simulink model "fir_simulation"  (R2012b)
settings: Solver=ode45  StartTime=0.0  StopTime=150000  RelTol=1e-3
values from neighbouring files (symbols this model uses):
  Fs = 640e6    (= 640000000)    [filter_coefficients.m]    (also in filter_design.m; filter_design_getting_order.m)
undefined symbols (not defined in the file or in its folder): get, sided, Two, xlipgetpartsetting
libraries: xbsIndex_r4 x7, dspsigops x5, dspsnks4 x5, dspspect3 x2, simulink x1, simulink_extras x1, casper_library_sources x1, xps_library x1
settings Model: Creator=heystek  LastModifiedBy=heystek

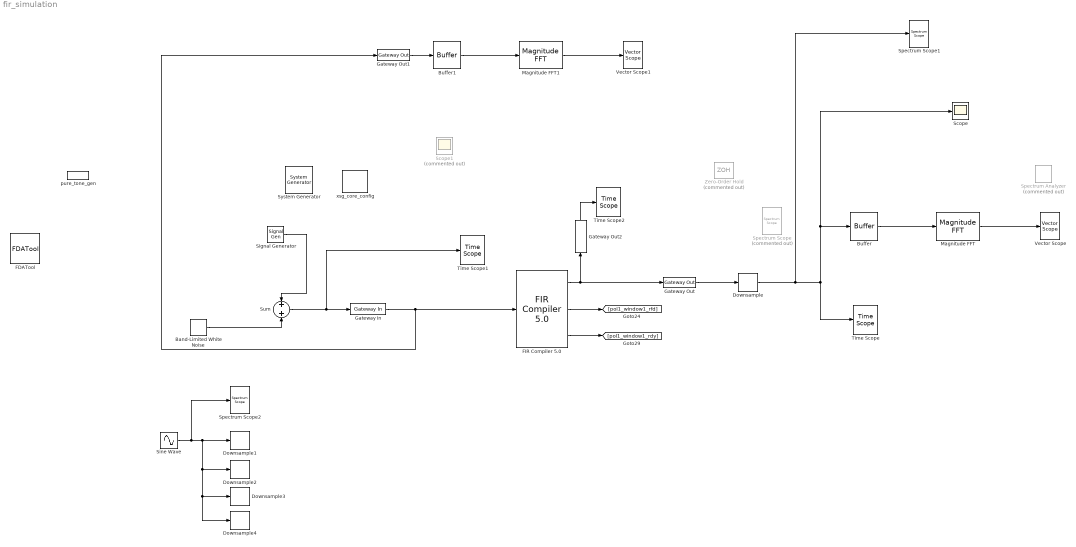
== system fir_simulation ==
  " System Generator" : xbsIndex_r4/ System Generator  Tag=genX  xilinxfamily=virtex6  part=xc6vsx475t  speed=-1  package=ff1759  synthesis_tool=XST  clock_wrapper=Clock Enables  directory=./window_design/sysgen  proj_type=Project Navigator  Synth_file=XST Defaults  Impl_file=ISE Defaults  testbench=off  simulink_period=1  sysclk_period=6.25  dcm_input_clock_period=100  incr_netlist=off  trim_vbits=Everywhere in SubSystem  dbl_ovrd=According to Block Masks  core_generation=According to Block Masks  run_coregen=off  deprecated_control=off  eval_field=0  block_type=sysgen
  Band-Limited White Noise : simulink/Sources/Band-Limited White Noise  Cov=[0.0]  Ts=0.25  seed=[23341]
  Buffer : Buffer  N=256  ic=20  TreatMby1Signals=One channel
  Buffer1 : Buffer  N=1024  TreatMby1Signals=One channel
  Downsample : dspsigops/Downsample  N=50  phase=0  RateOptions=Allow multirate processing  smode=Allow multirate  fmode=Maintain input frame size  ic=0
  Downsample1 : dspsigops/Downsample  N=4  phase=0  RateOptions=Allow multirate processing  smode=Allow multirate  fmode=Maintain input frame size  ic=0
  Downsample2 : dspsigops/Downsample  N=4  phase=1  RateOptions=Allow multirate processing  smode=Allow multirate  fmode=Maintain input frame size  ic=0
  Downsample3 : dspsigops/Downsample  N=4  phase=2  RateOptions=Allow multirate processing  smode=Allow multirate  fmode=Maintain input frame size  ic=0
  Downsample4 : dspsigops/Downsample  N=4  phase=3  RateOptions=Allow multirate processing  smode=Allow multirate  fmode=Maintain input frame size  ic=0
  FDATool : xbsIndex_r4/FDATool  block_type=fdatool
      settings: infoedit=FDATool
  "FIR Compiler 5.0 " : xbsIndex_r4/FIR Compiler 5.0   coefficientvector=coef  coefficient_sets=1  filter_type=Decimation  rate_change_type=Integer  interpolation_rate=1  decimation_rate=50  zero_pack_factor=1  number_channels=1  ratespecification=Maximum_Possible  sampleperiod=1  hardwareoversamplingrate=1  filter_architecture=Systolic_Multiply_Accumulate  coefficient_reload=off  coefficient_structure=Non_Symmetric  coefficient_sign=Unsigned  quantization=Maximize_Dynamic_Range  coefficient_width=16  bestprecision=on  coefficient_fractional_bits=24  number_paths=1  output_rounding_mode=Convergent_Rounding_to_Even  output_width=16  allow_rounding_approximation=off  optimization_goal=Area  has_sclr=off  has_data_valid=off  has_nd=off  has_ce=off  usechan_in_adv=off  chan_in_adv=0  data_buffer_type=Automatic  coefficient_buffer_type=Automatic  input_buffer_type=Automatic  output_buffer_type=Automatic  preference_for_other_storage=Automatic  multi_column_support=Disabled  columnconfig='12'  inter_column_pipe_length=4  passband_min=0.0  passband_max=0.5  stopband_min=0.5  stopband_max=1.0  filter_selection=1  gui_behaviour=Sysgen  registered_output=true  data_sign=Signed  data_width=16  data_fractional_bits=0  wrapper_available=true  ip_wrap_arbitrary_binary_point=true  ip_name=FIR Compiler  ip_version=5.0  dsptool_ready=true  ipcore_usecache=true  ipcore_useipmodelcache=true  ipcore_xco_need_fpga_part=true  port_translation_map={ 'ce' => 'en', 'sclr' => 'rst' }  run_core_at_system_period=true  ipcore_fpga_part=xlipgetpartsetting(gcb, {'virtex4', 'xc4vsx35', '-10', 'ff668'})  structural_sim=false  block_type=fir_compiler_v5_0
  Gateway In : xbsIndex_r4/Gateway In  gui_display_data_type=Fixed-point  arith_type="Signed  (2's comp)"  n_bits=16  bin_pt=16  preci_type=Single  exp_width=8  frac_width=24  quantization="Round  (unbiased: +/- Inf)"  overflow=Saturate  period=1  dbl_ovrd=off  timing_constraint=None  locs_specified=off  LOCs={}  UseAsADC=off  ADCChannel='1'  inherit_from_input=off  hdl_port=on  block_type=gatewayin
  Gateway Out : xbsIndex_r4/Gateway Out  inherit_from_input=on  hdl_port=off  timing_constraint=None  locs_specified=off  LOCs={}  UseAsDAC=off  DACChannel='1'  block_type=gatewayout
  Gateway Out1 : xbsIndex_r4/Gateway Out  inherit_from_input=off  hdl_port=on  timing_constraint=None  locs_specified=off  LOCs={}  UseAsDAC=off  DACChannel='1'  block_type=gatewayout
  Gateway Out2 : xbsIndex_r4/Gateway Out  inherit_from_input=off  hdl_port=on  timing_constraint=None  locs_specified=off  LOCs={}  UseAsDAC=off  DACChannel='1'  block_type=gatewayout
  Magnitude FFT : dspspect3/Magnitude FFT  mag_or_magsq=Magnitude squared  FFTImplementation=Auto  fftLenInherit=off  fftsize=256
  Magnitude FFT1 : dspspect3/Magnitude FFT  mag_or_magsq=Magnitude squared  FFTImplementation=Auto  fftLenInherit=off  fftsize=1024
  Scope : Scope
      settings: YMin=-0.00065  YMax=0.0002
  Scope1 : Scope  Commented=on
      settings: YMin=0.055  YMax=0.1
  Signal Generator : SignalGenerator  Amplitude=0.1  Frequency=0.00353  VectorParams1D=off
  Sine Wave : Sin  SineType=Sample based  Amplitude=0.1  Frequency=5  Samples=2048  SampleTime=0.25  Offset=1
  Spectrum Analyzer : simulink_extras/Additional Sinks/Spectrum Analyzer  Commented=on  npts=256  fftpts=256  HowOften=64  sampleT=0.1
  Spectrum Scope : dspsnks4/Spectrum Scope  Commented=on  ScopeProperties=on  Domain=Frequency  HorizSpan=1  UseBuffer=off  BufferSize=128  Overlap=0  TreatMby1Signals=One channel  inpFftLenInherit=on  FFTlength=128  numAvg=2  DisplayProperties=off  AxisGrid=on  Memory=off  FrameNumber=on  AxisLegend=off  AxisZoom=off  OpenScopeAtSimStart=on  OpenScopeImmediately=off  FigPos=get(0,'defaultfigureposition')  AxisProperties=off  XUnits=Hertz  XRange=Two-sided ((-Fs/2...Fs/2])  XDisplay=0  InheritXIncr=on  XIncr=1.0  XLabel=Samples  XLimit=Auto  YUnits=dBW/Hertz  XMax=1  XMin=0  YLabel=Magnitude-squared, dB  LineProperties=off  wintypeSpecScope=Hann  RsSpecScope=50  betaSpecScope=5  winsampSpecScope=Periodic  XAxisParamsVer=6.9  isFrameUpgraded=on
      settings: YMin=-10  YMax=10
  Spectrum Scope1 : dspsnks4/Spectrum Scope  ScopeProperties=on  Domain=Frequency  HorizSpan=1  UseBuffer=on  BufferSize=256  Overlap=0  TreatMby1Signals=One channel  inpFftLenInherit=on  FFTlength=256  numAvg=5  DisplayProperties=off  AxisGrid=on  Memory=off  FrameNumber=on  AxisLegend=off  AxisZoom=off  OpenScopeAtSimStart=on  OpenScopeImmediately=off  FigPos=get(0,'defaultfigureposition')  AxisProperties=off  XUnits=Hertz  XRange=Two-sided ((-Fs/2...Fs/2])  XDisplay=0  InheritXIncr=on  XIncr=1.0  XLabel=Samples  XLimit=Auto  YUnits=dBW/Hertz  XMax=1  XMin=0  YLabel=Magnitude-squared, dB  LineProperties=off  wintypeSpecScope=Hann  RsSpecScope=50  betaSpecScope=5  winsampSpecScope=Periodic  XAxisParamsVer=6.9  isFrameUpgraded=on
      settings: YMin=-10  YMax=10
  Spectrum Scope2 : dspsnks4/Spectrum Scope  ScopeProperties=on  Domain=Frequency  HorizSpan=1  UseBuffer=on  BufferSize=256  Overlap=0  TreatMby1Signals=One channel  inpFftLenInherit=on  FFTlength=256  numAvg=5  DisplayProperties=off  AxisGrid=on  Memory=off  FrameNumber=on  AxisLegend=off  AxisZoom=off  OpenScopeAtSimStart=on  OpenScopeImmediately=off  FigPos=get(0,'defaultfigureposition')  AxisProperties=off  XUnits=Hertz  XRange=Two-sided ((-Fs/2...Fs/2])  XDisplay=0  InheritXIncr=on  XIncr=1.0  XLabel=Samples  XLimit=Auto  YUnits=dBW/Hertz  XMax=1  XMin=0  YLabel=Magnitude-squared, dB  LineProperties=off  wintypeSpecScope=Hann  RsSpecScope=50  betaSpecScope=5  winsampSpecScope=Periodic  XAxisParamsVer=6.9  isFrameUpgraded=on
      settings: YMin=-10  YMax=10
  Sum : Sum
  Time Scope : TimeScope  DefaultConfigurationName=spbscopes.TimeScopeBlockCfg
      settings: CopyFcn=scopeextensions.ScopeBlock.callback(gcbh, 'onBlockCopy', gcbh);  DeleteFcn=scopeextensions.ScopeBlock.callback(gcbh, 'onBlockDelete');  PreSaveFcn=scopeextensions.ScopeBlock.callback(gcbh, 'onModelSave');  NameChangeFcn=scopeextensions.ScopeBlock.callback(gcbh, 'onBlockRename');  OpenFcn=scopeextensions.SrcWiredSL.coreBlockCommand('Open',gcbh)  CloseFcn=scopeextensions.ScopeBlock.callback(gcbh, 'onBlockClose');  PreDeleteFcn=scopeextensions.ScopeBlock.callback(gcbh, 'onBlockPreDelete');
  Time Scope1 : TimeScope  DefaultConfigurationName=spbscopes.TimeScopeBlockCfg
      settings: CopyFcn=scopeextensions.ScopeBlock.callback(gcbh, 'onBlockCopy', gcbh);  DeleteFcn=scopeextensions.ScopeBlock.callback(gcbh, 'onBlockDelete');  PreSaveFcn=scopeextensions.ScopeBlock.callback(gcbh, 'onModelSave');  NameChangeFcn=scopeextensions.ScopeBlock.callback(gcbh, 'onBlockRename');  OpenFcn=scopeextensions.SrcWiredSL.coreBlockCommand('Open',gcbh)  CloseFcn=scopeextensions.ScopeBlock.callback(gcbh, 'onBlockClose');  PreDeleteFcn=scopeextensions.ScopeBlock.callback(gcbh, 'onBlockPreDelete');
  Time Scope2 : TimeScope  DefaultConfigurationName=spbscopes.TimeScopeBlockCfg
      settings: CopyFcn=scopeextensions.ScopeBlock.callback(gcbh, 'onBlockCopy', gcbh);  DeleteFcn=scopeextensions.ScopeBlock.callback(gcbh, 'onBlockDelete');  PreSaveFcn=scopeextensions.ScopeBlock.callback(gcbh, 'onModelSave');  NameChangeFcn=scopeextensions.ScopeBlock.callback(gcbh, 'onBlockRename');  OpenFcn=scopeextensions.SrcWiredSL.coreBlockCommand('Open',gcbh)  CloseFcn=scopeextensions.ScopeBlock.callback(gcbh, 'onBlockClose');  PreDeleteFcn=scopeextensions.ScopeBlock.callback(gcbh, 'onBlockPreDelete');
  Vector Scope : dspsnks4/Vector Scope  ScopeProperties=on  Domain=Frequency  HorizSpan=1  DisplayProperties=off  AxisGrid=on  Memory=off  FrameNumber=on  AxisLegend=on  AxisZoom=off  OpenScopeAtSimStart=on  OpenScopeImmediately=off  FigPos=get(0,'defaultfigureposition')  AxisProperties=off  XUnits=Hertz  XRange=[-Fs/2...Fs/2]  InheritXIncr=on  XIncr=50  XLabel=Time  XLimit=Auto  XMin=-1e6  XMax=1e6  XStart=0  YUnits=dB  YLabel=Amplitude  LineProperties=off  XAxisParamsVer=6.9
      settings: YMin=-50  YMax=30
  Vector Scope1 : dspsnks4/Vector Scope  ScopeProperties=on  Domain=Frequency  HorizSpan=1  DisplayProperties=off  AxisGrid=on  Memory=off  FrameNumber=on  AxisLegend=on  AxisZoom=off  OpenScopeAtSimStart=on  OpenScopeImmediately=off  FigPos=get(0,'defaultfigureposition')  AxisProperties=off  XUnits=Hertz  XRange=[-Fs/2...Fs/2]  InheritXIncr=on  XIncr=1  XLabel=Time  XLimit=Auto  XMin=-1e6  XMax=1e6  XStart=0  YUnits=Magnitude  YLabel=Amplitude  LineProperties=off  XAxisParamsVer=6.9
      settings: YMin=-10  YMax=10
  Zero-Order Hold : ZeroOrderHold  Commented=on
  pure_tone_gen : casper_library_sources/pure_tone_gen  adc_demux_factor=8  num_fft_channels=1024  tone_channel=3
  xsg_core_config : xps_library/XSG_core_config  Tag=xps:xsg  hw_sys=ROACH2:sx475t  clk_src=sys_clk  ROACH_clk_src=adc0_clk  ROACH2_clk_src=sys_clk  MKDIG_clk_src=sys_clk  clk_rate=200  sample_period=1  synthesis_tool=XST
  wires:
  Band-Limited White Noise/1 -> Sum/2
  "FIR Compiler 5.0 "/2 -> [pol1_window1_rfd]
  "FIR Compiler 5.0 "/3 -> [pol1_window1_rdy]
  Gateway In/1 -> Gateway Out1/1, "FIR Compiler 5.0 "/1
  Gateway Out/1 -> Downsample/1
  Buffer/1 -> Magnitude FFT/1
  Magnitude FFT/1 -> Vector Scope/1
  Signal Generator/1 -> Sum/1
  Buffer1/1 -> Magnitude FFT1/1
  Magnitude FFT1/1 -> Vector Scope1/1
  Gateway Out1/1 -> Buffer1/1
  Sum/1 -> Time Scope1/1, Gateway In/1
  "FIR Compiler 5.0 "/1 -> Gateway Out/1, Gateway Out2/1
  Gateway Out2/1 -> Time Scope2/1
  Downsample/1 -> Spectrum Scope1/1, Scope/1, Buffer/1, Time Scope/1
  Sine Wave/1 -> Spectrum Scope2/1, Downsample4/1, Downsample3/1, Downsample2/1, Downsample1/1
